simulink model "trabalhofinal_vR2012a"  (R2012a)
settings: Solver=FixedStepDiscrete  StartTime=0.0  StopTime=0.5  FixedStep=0.1e-6  MaxStep=50e-6
undefined symbols (not defined in the file): DiscIntNeverNeededParam, Ipac0, Vpac0
libraries: powerlib x36, simulink x19, fuzblock x7, powerlib_extras x2, powerlib_meascontrol x2
(part 3 of 3)

== system trabalhofinal_vR2012a/PV array PI/DSOGI1/Calcula Impedância2/PLL ==
  Falbe : Inport
  wt : Inport  Port=2
  Constant1 : Constant  Value=wB
  Constant2 : Constant  Value=wB
  Gain : Gain  Gain=-1/Vp
  Integrator : Integrator  InitialCondition=phase0_v  UpperSaturationLimit=2*pi  LowerSaturationLimit=0
  Mux : Mux  Inputs=2
  Mux1 : Mux  Inputs=2
  PID Controller : simulink/Continuous/PID Controller  Controller=PI  TimeDomain=Continuous-time  SampleTime=-1  IntegratorMethod=Forward Euler  FilterMethod=Forward Euler  Form=Parallel  UseFilter=on  ControllerParametersSource=internal  P=kp_PLL  I=ki_PLL  D=0  N=100  InitialConditionSource=internal  InitialConditionForIntegrator=0  InitialConditionForFilter=0  ExternalReset=none  LimitOutput=off  UpperSaturationLimit=inf  LowerSaturationLimit=-inf  LinearizeAsGain=on  AntiWindupMode=none  Kb=1  TrackingMode=off  Kt=1  PParamMin=[]  PParamMax=[]  IParamMin=[]  IParamMax=[]  DParamMin=[]  DParamMax=[]  NParamMin=[]  NParamMax=[]  KbParamMin=[]  KbParamMax=[]  KtParamMin=[]  KtParamMax=[]  POutMin=[]  POutMax=[]  IOutMin=[]  IOutMax=[]  DOutMin=[]  DOutMax=[]  NOutMin=[]  NOutMax=[]  KbOutMin=[]  KbOutMax=[]  KtOutMin=[]  KtOutMax=[]  IntegratorOutMin=[]  IntegratorOutMax=[]  FilterOutMin=[]  FilterOutMax=[]  SumOutMin=[]  SumOutMax=[]  SumI1OutMin=[]  SumI1OutMax=[]  SumI2OutMin=[]  SumI2OutMax=[]  SumI3OutMin=[]  SumI3OutMax=[]  SumDOutMin=[]  SumDOutMax=[]  SaturationOutMin=[]  SaturationOutMax=[]  IntegratorContinuousStateAttributes=''  IntegratorStateMustResolveToSignalObject=off  IntegratorRTWStateStorageClass=Auto  FilterContinuousStateAttributes=''  FilterStateMustResolveToSignalObject=off  FilterRTWStateStorageClass=Auto  DifferentiatorICPrevScaledInput=0  DifferentiatorOutMin=[]  DifferentiatorOutMax=[]
  PLL : Scope  NumInputPorts=4
      settings: TimeRange=auto  MaxDataPoints=5000  SaveToWorkspace=off  SaveName=ScopeData  YMin=-1.75~-0.25~7~368  YMax=1.75~1.75~15~377  SampleTime=-1
  Sum2 : Sum  Inputs=|++
  abc2dq0 PSIM : Subsystem
  Fqd : Outport
  w : Outport  Port=2
  ro : Outport  Port=3
  wires:
  wt/1 -> abc2dq0 PSIM/2(wt)
  [w] -> Mux1/1  "w"
  Integrator/1 -> [ro], ro/1
  abc2dq0 PSIM/2(Fd) -> Gain/1, Mux/2
  [Falbe] -> PLL/1  "Falbe"
  Falbe/1 -> [Falbe], abc2dq0 PSIM/1(Falbe)
  [ro] -> PLL/3  "ro"
  [Fqd] -> PLL/2  "Fqd"
  Constant2/1 -> Sum2/2
  Mux/1 -> Fqd/1, [Fqd]
  abc2dq0 PSIM/1(Fq) -> Mux/1
  Sum2/1 -> Integrator/1, w/1, [w]
  Gain/1 -> PID Controller/1
  Mux1/1 -> PLL/4
  Constant1/1 -> Mux1/2
  PID Controller/1 -> Sum2/1

== system trabalhofinal_vR2012a/PV array PI/DSOGI1/Calcula Impedância2/abc2albe ==
  Fabc : Inport
  Gain1 : Gain  Gain=2/3  SaturateOnIntegerOverflow=on  OutDataTypeStr=Inherit: Same as input  ParamDataTypeStr=Inherit: Same as input
  Gain3 : Gain  Gain="[ 1   -1/2   -1/2; 0   sqrt(3)/2   -sqrt(3)/2 ]"  Multiplication=Matrix(K*u) (u vector)  SaturateOnIntegerOverflow=on  OutDataTypeStr=Inherit: Same as input  ParamDataTypeStr=Inherit: Same as input
  Falbe : Outport
  wires:
  Gain1/1 -> Falbe/1
  Gain3/1 -> Gain1/1
  Fabc/1 -> Gain3/1

== system trabalhofinal_vR2012a/PV array PI/DSOGI1/Calcula Impedância2/abc2albe1 ==
  Fabc : Inport
  Gain1 : Gain  Gain=2/3  SaturateOnIntegerOverflow=on  OutDataTypeStr=Inherit: Same as input  ParamDataTypeStr=Inherit: Same as input
  Gain3 : Gain  Gain="[ 1   -1/2   -1/2; 0   sqrt(3)/2   -sqrt(3)/2 ]"  Multiplication=Matrix(K*u) (u vector)  SaturateOnIntegerOverflow=on  OutDataTypeStr=Inherit: Same as input  ParamDataTypeStr=Inherit: Same as input
  Falbe : Outport
  wires:
  Fabc/1 -> Gain3/1
  Gain3/1 -> Gain1/1
  Gain1/1 -> Falbe/1

== system trabalhofinal_vR2012a/PV array PI/DSOGI1/Calcula Impedância2/abc2dq0 PSIM ==
  Falbe : Inport
  wt : Inport  Port=2
  Fcn1 : Fcn  Expr=u(1)*cos(u(3))+u(2)*sin(u(3))
  Fcn2 : Fcn  Expr=u(1)*sin(u(3))-u(2)*cos(u(3))
  Mux : Mux  Inputs=2
  Mux1 : Mux  Inputs=2
  Fqd : Outport
  wires:
  Mux1/1 -> Fqd/1
  Mux/1 -> Fcn1/1, Fcn2/1
  wt/1 -> Mux/2
  Fcn2/1 -> Mux1/2
  Fcn1/1 -> Mux1/1
  Falbe/1 -> Mux/1

== system trabalhofinal_vR2012a/PV array Fuzzy/DSOGI1/Calcula Impedância2/DSOGI (Corrente)/SOGI BPF (beta) ==
  wr : Inport
  fbe : Inport  Port=2
  Gain : Gain  Gain=1/2
  Gain2 : Gain  Gain=k
  Integrator : Integrator  InitialCondition=int3_i
  Integrator1 : Integrator  InitialCondition=int4_i
  Product : Product
  Product1 : Product
  Sum : Sum  Inputs=-+|
  Sum2 : Sum  Inputs=|+-
  fbe' : Outport
  qfbe' : Outport  Port=2
  wires:
  fbe/1 -> Gain/1
  Gain/1 -> Sum/2
  Product/1 -> Integrator/1
  Gain2/1 -> Sum2/1
  Integrator/1 -> Product1/2, Sum/1, fbe'/1
  Product1/1 -> Integrator1/1
  Sum/1 -> Gain2/1
  Sum2/1 -> Product/2
  wr/1 -> Product/1, Product1/1
  Integrator1/1 -> Sum2/2, qfbe'/1

== system trabalhofinal_vR2012a/PV array Fuzzy/DSOGI1/Calcula Impedância2/DSOGI (Corrente)/SOGI BPF(alfa)  ==
  wr : Inport
  fal : Inport  Port=2
  Gain : Gain  Gain=1/2
  Gain2 : Gain  Gain=k
  Integrator : Integrator  InitialCondition=int1_i
  Integrator1 : Integrator  InitialCondition=int2_i
  Product : Product
  Product1 : Product
  Sum : Sum  Inputs=-+|
  Sum2 : Sum  Inputs=|+-
  fal' : Outport
  qfal' : Outport  Port=2
  wires:
  Integrator1/1 -> qfal'/1, Sum2/2
  wr/1 -> Product1/1, Product/1
  Sum2/1 -> Product/2
  Sum/1 -> Gain2/1
  Product1/1 -> Integrator1/1
  Integrator/1 -> fal'/1, Sum/1, Product1/2
  Gain2/1 -> Sum2/1
  Product/1 -> Integrator/1
  Gain/1 -> Sum/2
  fal/1 -> Gain/1

== system trabalhofinal_vR2012a/PV array Fuzzy/DSOGI1/Calcula Impedância2/DSOGI (Tensão)/SOGI BPF (beta) ==
  wr : Inport
  fbe : Inport  Port=2
  Gain : Gain  Gain=1/2
  Gain2 : Gain  Gain=k
  Integrator : Integrator  InitialCondition=int3_v
  Integrator1 : Integrator  InitialCondition=int4_v
  Product : Product
  Product1 : Product
  Sum : Sum  Inputs=-+|
  Sum2 : Sum  Inputs=|+-
  fbe' : Outport
  qfbe' : Outport  Port=2
  wires:
  fbe/1 -> Gain/1
  Gain/1 -> Sum/2
  Product/1 -> Integrator/1
  Gain2/1 -> Sum2/1
  Integrator/1 -> Product1/2, Sum/1, fbe'/1
  Product1/1 -> Integrator1/1
  Sum/1 -> Gain2/1
  Sum2/1 -> Product/2
  wr/1 -> Product/1, Product1/1
  Integrator1/1 -> Sum2/2, qfbe'/1

== system trabalhofinal_vR2012a/PV array Fuzzy/DSOGI1/Calcula Impedância2/DSOGI (Tensão)/SOGI BPF(alfa)  ==
  wr : Inport
  fal : Inport  Port=2
  Gain : Gain  Gain=1/2
  Gain2 : Gain  Gain=k
  Integrator : Integrator  InitialCondition=int1_v
  Integrator1 : Integrator  InitialCondition=int2_v
  Product : Product
  Product1 : Product
  Sum : Sum  Inputs=-+|
  Sum2 : Sum  Inputs=|+-
  fal' : Outport
  qfal' : Outport  Port=2
  wires:
  Integrator1/1 -> qfal'/1, Sum2/2
  wr/1 -> Product1/1, Product/1
  Sum2/1 -> Product/2
  Sum/1 -> Gain2/1
  Product1/1 -> Integrator1/1
  Integrator/1 -> fal'/1, Sum/1, Product1/2
  Gain2/1 -> Sum2/1
  Product/1 -> Integrator/1
  Gain/1 -> Sum/2
  fal/1 -> Gain/1

== system trabalhofinal_vR2012a/PV array Fuzzy/DSOGI1/Calcula Impedância2/PLL/abc2dq0 PSIM ==
  Falbe : Inport
  wt : Inport  Port=2
  Fcn1 : Fcn  Expr=u(1)*cos(u(3))+u(2)*sin(u(3))
  Fcn2 : Fcn  Expr=u(1)*sin(u(3))-u(2)*cos(u(3))
  Mux : Mux  Inputs=2
  Fq : Outport
  Fd : Outport  Port=2
  wires:
  Mux/1 -> Fcn1/1, Fcn2/1
  wt/1 -> Mux/2
  Fcn2/1 -> Fd/1
  Fcn1/1 -> Fq/1
  Falbe/1 -> Mux/1

== system trabalhofinal_vR2012a/PV array PI/DSOGI1/Calcula Impedância2/DSOGI (Corrente)/SOGI BPF (beta) ==
  wr : Inport
  fbe : Inport  Port=2
  Gain : Gain  Gain=1/2
  Gain2 : Gain  Gain=k
  Integrator : Integrator  InitialCondition=int3_i
  Integrator1 : Integrator  InitialCondition=int4_i
  Product : Product
  Product1 : Product
  Sum : Sum  Inputs=-+|
  Sum2 : Sum  Inputs=|+-
  fbe' : Outport
  qfbe' : Outport  Port=2
  wires:
  fbe/1 -> Gain/1
  Gain/1 -> Sum/2
  Product/1 -> Integrator/1
  Gain2/1 -> Sum2/1
  Integrator/1 -> Product1/2, Sum/1, fbe'/1
  Product1/1 -> Integrator1/1
  Sum/1 -> Gain2/1
  Sum2/1 -> Product/2
  wr/1 -> Product/1, Product1/1
  Integrator1/1 -> Sum2/2, qfbe'/1

== system trabalhofinal_vR2012a/PV array PI/DSOGI1/Calcula Impedância2/DSOGI (Corrente)/SOGI BPF(alfa)  ==
  wr : Inport
  fal : Inport  Port=2
  Gain : Gain  Gain=1/2
  Gain2 : Gain  Gain=k
  Integrator : Integrator  InitialCondition=int1_i
  Integrator1 : Integrator  InitialCondition=int2_i
  Product : Product
  Product1 : Product
  Sum : Sum  Inputs=-+|
  Sum2 : Sum  Inputs=|+-
  fal' : Outport
  qfal' : Outport  Port=2
  wires:
  Integrator1/1 -> qfal'/1, Sum2/2
  wr/1 -> Product1/1, Product/1
  Sum2/1 -> Product/2
  Sum/1 -> Gain2/1
  Product1/1 -> Integrator1/1
  Integrator/1 -> fal'/1, Sum/1, Product1/2
  Gain2/1 -> Sum2/1
  Product/1 -> Integrator/1
  Gain/1 -> Sum/2
  fal/1 -> Gain/1

== system trabalhofinal_vR2012a/PV array PI/DSOGI1/Calcula Impedância2/DSOGI (Tensão)/SOGI BPF (beta) ==
  wr : Inport
  fbe : Inport  Port=2
  Gain : Gain  Gain=1/2
  Gain2 : Gain  Gain=k
  Integrator : Integrator  InitialCondition=int3_v
  Integrator1 : Integrator  InitialCondition=int4_v
  Product : Product
  Product1 : Product
  Sum : Sum  Inputs=-+|
  Sum2 : Sum  Inputs=|+-
  fbe' : Outport
  qfbe' : Outport  Port=2
  wires:
  fbe/1 -> Gain/1
  Gain/1 -> Sum/2
  Product/1 -> Integrator/1
  Gain2/1 -> Sum2/1
  Integrator/1 -> Product1/2, Sum/1, fbe'/1
  Product1/1 -> Integrator1/1
  Sum/1 -> Gain2/1
  Sum2/1 -> Product/2
  wr/1 -> Product/1, Product1/1
  Integrator1/1 -> Sum2/2, qfbe'/1

== system trabalhofinal_vR2012a/PV array PI/DSOGI1/Calcula Impedância2/DSOGI (Tensão)/SOGI BPF(alfa)  ==
  wr : Inport
  fal : Inport  Port=2
  Gain : Gain  Gain=1/2
  Gain2 : Gain  Gain=k
  Integrator : Integrator  InitialCondition=int1_v
  Integrator1 : Integrator  InitialCondition=int2_v
  Product : Product
  Product1 : Product
  Sum : Sum  Inputs=-+|
  Sum2 : Sum  Inputs=|+-
  fal' : Outport
  qfal' : Outport  Port=2
  wires:
  Integrator1/1 -> qfal'/1, Sum2/2
  wr/1 -> Product1/1, Product/1
  Sum2/1 -> Product/2
  Sum/1 -> Gain2/1
  Product1/1 -> Integrator1/1
  Integrator/1 -> fal'/1, Sum/1, Product1/2
  Gain2/1 -> Sum2/1
  Product/1 -> Integrator/1
  Gain/1 -> Sum/2
  fal/1 -> Gain/1

== system trabalhofinal_vR2012a/PV array PI/DSOGI1/Calcula Impedância2/PLL/abc2dq0 PSIM ==
  Falbe : Inport
  wt : Inport  Port=2
  Fcn1 : Fcn  Expr=u(1)*cos(u(3))+u(2)*sin(u(3))
  Fcn2 : Fcn  Expr=u(1)*sin(u(3))-u(2)*cos(u(3))
  Mux : Mux  Inputs=2
  Fq : Outport
  Fd : Outport  Port=2
  wires:
  Mux/1 -> Fcn1/1, Fcn2/1
  wt/1 -> Mux/2
  Fcn2/1 -> Fd/1
  Fcn1/1 -> Fq/1
  Falbe/1 -> Mux/1
